simulink model "Prac3_carro"  (R2025a)
settings: Solver=ode45  StartTime=0.0  StopTime=10  RelTol=1e-3
values from neighbouring files (symbols this model uses):
  b1 = 1000    [main_prac3.m]    (also in prac3.m)
  f = 0    [main_prac3.m]    (also in prac3.m)
  k1 = 16182    [main_prac3.m]    (also in prac3.m)
  k2 = 19000    [main_prac3.m]    (also in prac3.m)
  m1 = 290    [main_prac3.m]    (also in prac3.m)
  m2 = 59    [main_prac3.m]    (also in prac3.m)
undefined symbols (not defined in the file or in its folder): w1, w2, x1_0, x2_0, xd1_0, xd2_0, z1_0, z2_0, zd1_0, zd2_0

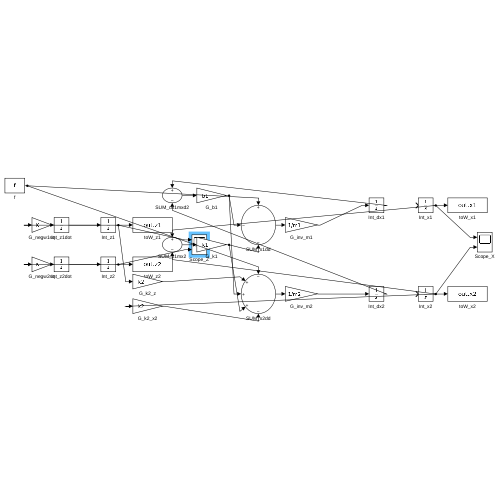
[thumbnail: Simulink's stored preview of the top-level diagram]
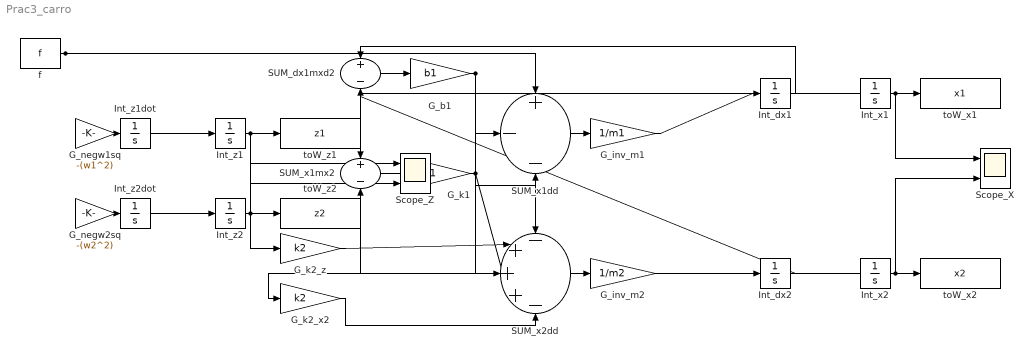
== system Prac3_carro ==
  G_b1 : Gain  Gain=b1
  G_inv_m1 : Gain  Gain=1/m1
  G_inv_m2 : Gain  Gain=1/m2
  G_k1 : Gain  Gain=k1
  G_k2_x2 : Gain  Gain=k2
  G_k2_z : Gain  Gain=k2
  G_negw1sq : Gain  Gain=-(w1^2)
  G_negw2sq : Gain  Gain=-(w2^2)
  Int_dx1 : Integrator  InitialCondition=xd1_0
  Int_dx2 : Integrator  InitialCondition=xd2_0
  Int_x1 : Integrator  InitialCondition=x1_0
  Int_x2 : Integrator  InitialCondition=x2_0
  Int_z1 : Integrator  InitialCondition=z1_0
  Int_z1dot : Integrator  InitialCondition=zd1_0
  Int_z2 : Integrator  InitialCondition=z2_0
  Int_z2dot : Integrator  InitialCondition=zd2_0
  SUM_dx1mxd2 : Sum  Inputs=+-
  SUM_x1dd : Sum  Inputs=+--
  SUM_x1mx2 : Sum  Inputs=+-
  SUM_x2dd : Sum  Inputs=-+++-
  Scope_X : Scope  NumInputPorts=2
      settings: ActiveDisplayYMinimum=-1.984367055836503  ActiveDisplayYMaximum=1.6073455962077574
  Scope_Z : Scope  NumInputPorts=2
      settings: ActiveDisplayYMinimum=-0.16885133135888031  ActiveDisplayYMaximum=0.15345286770227162
  f : Constant  Value=f
  toW_x1 : ToWorkspace  VariableName=x1  SaveFormat=Structure With Time  SampleTime=-1
  toW_x2 : ToWorkspace  VariableName=x2  SaveFormat=Structure With Time  SampleTime=-1
  toW_z1 : ToWorkspace  VariableName=z1  SaveFormat=Structure With Time  SampleTime=-1
  toW_z2 : ToWorkspace  VariableName=z2  SaveFormat=Structure With Time  SampleTime=-1
  wires:
  Int_z1/1 -> G_negw1sq/1, toW_z1/1, Scope_Z/1, G_k2_z/1
  G_negw1sq/1 -> Int_z1dot/1
  Int_z1dot/1 -> Int_z1/1
  Int_z2/1 -> G_negw2sq/1, toW_z2/1, Scope_Z/2
  G_negw2sq/1 -> Int_z2dot/1
  Int_z2dot/1 -> Int_z2/1
  Int_dx1/1 -> SUM_dx1mxd2/1
  Int_dx2/1 -> SUM_dx1mxd2/2
  Int_x1/1 -> SUM_x1mx2/1, Scope_X/1, toW_x1/1
  Int_x2/1 -> SUM_x1mx2/2, G_k2_x2/1, Scope_X/2, toW_x2/1
  SUM_dx1mxd2/1 -> G_b1/1
  SUM_x1mx2/1 -> G_k1/1
  f/1 -> SUM_x1dd/1, SUM_x2dd/1
  G_b1/1 -> SUM_x1dd/2, SUM_x2dd/3
  G_k1/1 -> SUM_x1dd/3, SUM_x2dd/4
  SUM_x1dd/1 -> G_inv_m1/1
  G_inv_m1/1 -> Int_dx1/1
  G_k2_z/1 -> SUM_x2dd/2
  G_k2_x2/1 -> SUM_x2dd/5
  SUM_x2dd/1 -> G_inv_m2/1
  G_inv_m2/1 -> Int_dx2/1
